simulink library "ddm"  (R2021b)
settings: Solver=VariableStepAuto  StartTime=0.0  StopTime=10.0  RelTol=1e-3
undefined symbols (not defined in the file or in its folder): ENUM_ADASACCSTA_ERROR, ENUM_ADASACCSTA_OFF, ENUM_ADASACCSTA_STANDBY, ENUM_ADASISASTA_OFF, ENUM_ALLOWMOV_ALLOWREADY, ENUM_APS, ENUM_BRKSTA_ERROR, ENUM_BRKSTA_OFF, ENUM_BRKSTA_ON, ENUM_CHGPREACTERRSTA_OBCPRE, ENUM_DCDCFAULTSTA_ANYFAULTLV1, ENUM_DCDCFAULTSTA_ANYFAULTLV2, ENUM_DRIVETRAIN_AWD, ENUM_DRIVETRAIN_FWD, ENUM_DRIVETRAIN_RWD, ENUM_DRSEATSTA_INVALID, ENUM_EDUDRTSTA_NORMAL, ENUM_EPBSTA_APPLIED, ENUM_EPBSTA_RELEASED, ENUM_HVBATTREADYPRE_READY, ENUM_MCUWARN_LV0, ENUM_MCUWARN_LV1, ENUM_MCUWARN_LV2, ENUM_MCUWARN_LV3, ENUM_MCUWARN_NOERROR, ENUM_OBCFAULTSTA_ANYFAULT, ENUM_PAS_R2F2, ENUM_PDFAULT_BATTPDFAIL, ENUM_PDFAULT_DCDCDISABLE, ENUM_PDFAULT_MCUDISABLE, ENUM_PDFAULT_MCUDISCHRG, ENUM_POWERSTA_OFF, ENUM_POWERSTA_ON, ENUM_POWERSTA_READY, ENUM_POWERSTA_STANDBY, ENUM_PRESSINDI_LOW, ENUM_PUFAULT_BATTUPFAIL, ENUM_PUFAULT_DCDCENABLEFAIL, ENUM_PUFAULT_PRECHRGCHKFAIL, ENUM_PUFAULT_SAFETYCHKFAIL, ENUM_PUSTATE_COMPLETED, ENUM_PWRSTASW_OFF, ENUM_PWRSTASW_OFFA, ENUM_PWRSTASW_OFFCHVCHRG, ENUM_PWRSTASW_OFFCLVCHRG, ENUM_PWRSTASW_ON, ENUM_PWRSTASW_ONHVCHRG, ENUM_PWRSTASW_READY, ENUM_PWRSTASW_STANDBY, ENUM_RANGESTA_12IN, ENUM_RANGESTA_12OUT, ENUM_SHIFTCOMMAND_D, ENUM_SHIFTCOMMAND_N, ENUM_SHIFTCOMMAND_P, ENUM_SHIFTCOMMAND_R, ENUM_ZONEMALFUNLV_1ST, ENUM_ZONEMALFUNLV_2ND, ENUM_ZONEMALFUNLV_3RD, ENUM_ZONEMALFUNLV_4TH, ENUM_ZONESPDCTRLMODE_ACC ... (+832)
libraries: hcu_lib x738, $bdroot x26, simulink x7
(part 21 of 25)

== system ddm/DDM/DDM/VMC_DDM/CCU Signal Error/CCU Signal Error  ==
  note: Fail Safe During Detection
  note: Test Detection Criteria
  note: Test Pass Criteria
  note: Release Condiction After Decision
  note: Release Condiction During Detection
  note: Fail Safe After Decision
  note: Diagnostics and Fault Handling
  task_time_s : Inport
  VDDM_C3CCU2LCCFS_flg : Inport  Port=2
  VDDM_C3CCU2RCCFS_flg : Inport  Port=3
  VDDM_C3CCU2CSCFS_flg : Inport  Port=4
  No_CAN_BUS_OFF : Inport  Port=5
  VPMM_PowerSta_enum : Inport  Port=6
  VINP_DCDCFaultSta_enum : Inport  Port=7
  DTC_clear_request : Inport  Port=8
  Constant : Constant  Value=ENUM_POWERSTA_OFF
  Constant1 : Constant  Value=ENUM_POWERSTA_OFF
  Constant{2,10,15,21,23} (5 alike) : Constant  Value=FALSE
  Constant11 : Constant  Value=KDDM_CCUSigErrPassSW_flg
  Constant12 : Constant  Value=ENUM_POWERSTA_OFF
  Constant13 : Constant  Value=ENUM_POWERSTA_STANDBY
  Constant{5,14,18,22} (4 alike) : Constant  Value=TRUE
  Constant3 : Constant  Value=ENUM_DCDCFAULTSTA_ANYFAULTLV2
  Constant33 : Constant  Value=KDDM_CCUSigErrDetSW_flg
  Constant34 : Constant  Value=KDDM_CCUSigErrDTC_cnt
  Constant35 : Constant  Value=KDDM_CCUSigErrCFSSW_flg
  Constant36 : Constant  Value=KDDM_CCUSigErrDFSSW_flg
  Constant4 : Constant  Value=KDDM_CCUSigErrDetTO_ms
  Constant6 : Constant  Value=KDDM_CCUSigErrPassTO_ms
  Constant7 : Constant  Value=KDDM_CCUSigErrDTC_cnt
  Constant8 : Constant  Value=ENUM_DCDCFAULTSTA_ANYFAULTLV2
  Constant9 : Constant  Value=KDDM_CCUSigErrPassTO_ms
  DTC_Couter : hcu_lib/Basic_Blocks/DTC_Couter
  DTC_Info : hcu_lib/Basic_Blocks/DTC_Info
  Data Type Conversion1 : DataTypeConversion  OutDataTypeStr=uint8
  Display1 : Display
  Display2 : Display
  Equal : RelationalOperator  Operator=~=  OutDataTypeStr=boolean  RndMeth=Simplest
  Equal1 : RelationalOperator  Operator=~=  OutDataTypeStr=boolean  RndMeth=Simplest
  Equal{2,4,6..7} (4 alike) : RelationalOperator  Operator===  OutDataTypeStr=boolean  RndMeth=Simplest
  Equal3 : RelationalOperator  OutDataTypeStr=boolean  RndMeth=Simplest
  From1 : From  Commented=on  GotoTag=VDDM_CCUSigErrDFS_flg
  Gain : Gain  Gain=XX2KXX
  Gain1 : Gain  Gain=KXX2XX
  Goto7 : Goto  Commented=on  GotoTag=VDDM_EDriveSysErrVCUErr_flg
  Logical Operator{3,5,9,15,19} (5 alike) : Logic  AllPortsSameDT=off  OutDataTypeStr=boolean
  Logical Operator{6,17..18,20..22,24} (7 alike) : Logic  Operator=NOT  AllPortsSameDT=off  OutDataTypeStr=boolean
  Logical Operator2 : Logic  Inputs=5  AllPortsSameDT=off  OutDataTypeStr=boolean
  Logical Operator23 : Logic  Inputs=5  AllPortsSameDT=off  OutDataTypeStr=boolean
  Logical Operator25 : Logic  Operator=OR  AllPortsSameDT=off  OutDataTypeStr=boolean
  Logical Operator7 : Logic  Operator=OR  AllPortsSameDT=off  OutDataTypeStr=boolean
  Logical Operator8 : Logic  Operator=OR  Inputs=3  AllPortsSameDT=off  OutDataTypeStr=boolean
  Relay : Relay  OnSwitchValue=ONE_INT  OffSwitchValue=ZERO_INT
  SR_Latch1 : hcu_lib/Basic_Blocks/SR_Latch
  SR_Latch4 : hcu_lib/Basic_Blocks/SR_Latch
  SR_Latch5 : hcu_lib/Basic_Blocks/SR_Latch
  Switch{,1..5} (6 alike) : Switch  Criteria=u2 ~= 0
  Terminator1 : Terminator
  Test Detection Criteria : hcu_lib/Basic_Blocks/Test Detection Criteria
  Timer1 : hcu_lib/Basic_Blocks/Timer
  Unit Delay2 : UnitDelay  SampleTime=-1  HasFrameUpgradeWarning=on
  VDDM_CCUSigErrCFS_flg : Outport
  VDDM_CCUSigErrDetDTC_raw32 : Outport  Port=2
  wires:
  Switch2/1 -> [VDDM_xxx_flg], Switch5/3
  Constant23/1 -> Switch1/3
  Constant22/1 -> Switch1/1
  Switch1/1 -> [VDDM_CCUSigErrDFSRls_flg]
  Constant21/1 -> Switch/3
  Switch/1 -> Goto7/1, Display1/1
  Constant18/1 -> Switch/1
  [VDDM_CCUSigErrCFS_flg] -> Switch/2
  [VDDM_CCUSigErrPass_flg] -> Switch1/2
  SR_Latch1/1 -> [VDDM_CCUSigErrPass_flg]
  From1/1 -> Terminator1/1
  [VDDM_CCUSigErrCFS_flg] -> VDDM_CCUSigErrCFS_flg/1
  Constant15/1 -> Switch4/3
  Equal3/1 -> SR_Latch1/1
  [task_time_s] -> Gain1/1
  Equal6/1 -> Logical Operator9/1
  Equal7/1 -> Logical Operator9/2
  Constant6/1 -> Equal3/2
  [VPMM_PowerSta_enum] -> Unit Delay2/1
  Logical Operator9/1 -> Logical Operator8/2
  Switch4/1 -> [VDDM_CCUSigErrCFSRls_flg], Display2/1
  [No_CAN_BUS_OFF] -> Logical Operator2/1
  [VDDM_CCUSigErrPass_flg] -> Logical Operator8/1
  [VDDM_xxx_flg] -> SR_Latch1/2
  [DTC_clear_request] -> Logical Operator8/3
  Logical Operator2/1 -> Switch2/2
  Logical Operator6/1 -> Timer1/1
  Constant13/1 -> Equal7/2
  Constant/1 -> Equal/2
  Unit Delay2/1 -> Equal6/1
  Constant12/1 -> Equal6/2
  Constant2/1 -> Switch2/3
  Constant14/1 -> Switch4/1
  [VPMM_PowerSta_enum] -> Equal7/1
  Logical Operator8/1 -> Switch4/2
  [VPMM_PowerSta_enum] -> Equal/1
  Timer1/1 -> Equal3/1
  VDDM_C3CCU2LCCFS_flg/1 -> [VDDM_C3CCU2LCCFS_flg]
  DTC_clear_request/1 -> [DTC_clear_request]
  VDDM_C3CCU2RCCFS_flg/1 -> [VDDM_C3CCU2RCCFS_flg]
  VPMM_PowerSta_enum/1 -> [VPMM_PowerSta_enum]
  VDDM_C3CCU2CSCFS_flg/1 -> [VDDM_C3CCU2CSCFS_flg]
  No_CAN_BUS_OFF/1 -> [No_CAN_BUS_OFF]
  VINP_DCDCFaultSta_enum/1 -> [VINP_DCDCFaultSta_enum]
  Equal/1 -> Logical Operator2/5
  [VDDM_C3CCU2LCCFS_flg] -> Logical Operator17/1
  [VDDM_C3CCU2RCCFS_flg] -> Logical Operator18/1
  [VDDM_C3CCU2CSCFS_flg] -> Logical Operator20/1
  [VINP_DCDCFaultSta_enum] -> Equal2/1
  Logical Operator17/1 -> Logical Operator2/2
  Logical Operator18/1 -> Logical Operator2/3
  Logical Operator20/1 -> Logical Operator2/4
  Logical Operator22/1 -> Logical Operator23/3
  [VDDM_C3CCU2LCCFS_flg] -> Logical Operator21/1
  [VPMM_PowerSta_enum] -> Equal1/1
  Logical Operator23/1 -> Switch3/2
  Constant5/1 -> Switch3/3
  Equal1/1 -> Logical Operator23/5
  [VDDM_C3CCU2RCCFS_flg] -> Logical Operator22/1
  Logical Operator24/1 -> Logical Operator23/4
  Logical Operator21/1 -> Logical Operator23/2
  [VDDM_C3CCU2CSCFS_flg] -> Logical Operator24/1
  [No_CAN_BUS_OFF] -> Logical Operator23/1
  Constant1/1 -> Equal1/2
  Switch3/1 -> Timer1/2, Logical Operator6/1
  task_time_s/1 -> [task_time_s]  "task_time_s"
  [task_time_s] -> Test Detection Criteria/2
  Constant4/1 -> Gain/1
  Gain/1 -> Test Detection Criteria/4
  Constant7/1 -> Test Detection Criteria/3
  Test Detection Criteria/1 -> [VDDM_CCUSigErrDet_flg]
  Gain1/1 -> Timer1/3
  Constant9/1 -> Timer1/4
  [VDDM_CCUSigErrCFSRls_flg] -> Logical Operator25/2
  [VDDM_CCUSigErrPass_flg] -> Logical Operator25/1
  Logical Operator7/1 -> SR_Latch4/2
  DTC_Couter/2 -> Data Type Conversion1/1
  Relay/1 -> SR_Latch4/1
  Logical Operator3/1 -> [VDDM_CCUSigErrDFS_flg]
  DTC_Couter/1 -> SR_Latch5/1
  Logical Operator25/1 -> Logical Operator15/1
  Constant11/1 -> Logical Operator15/2
  Constant36/1 -> Logical Operator3/1
  Constant34/1 -> DTC_Couter/3
  [VDDM_CCUSigErrDet_flg] -> Logical Operator19/1
  Logical Operator15/1 -> DTC_Couter/2
  Logical Operator19/1 -> DTC_Couter/1
  SR_Latch4/1 -> Logical Operator3/2
  [VDDM_CCUSigErrDTC_cnt] -> Relay/1
  Data Type Conversion1/1 -> [VDDM_CCUSigErrDTC_cnt]
  SR_Latch5/1 -> Logical Operator5/1
  Logical Operator5/1 -> [VDDM_CCUSigErrCFS_flg]
  [VDDM_CCUSigErrCFSRls_flg] -> SR_Latch5/2
  Constant35/1 -> Logical Operator5/2
  [VDDM_CCUSigErrDFSRls_flg] -> Logical Operator7/1
  Constant33/1 -> Logical Operator19/2
  [VDDM_CCUSigErrCFS_flg] -> Logical Operator7/2
  Constant3/1 -> Equal2/2
  Equal2/1 -> Switch2/1
  [VINP_DCDCFaultSta_enum] -> Equal4/1
  Constant8/1 -> Equal4/2
  Equal4/1 -> Switch3/1
  [DTC_clear_request] -> Switch5/2
  Constant10/1 -> Switch5/1
  Switch5/1 -> Test Detection Criteria/1
  [VDDM_CCUSigErrDet_flg] -> DTC_Info/1
  [VDDM_CCUSigErrPass_flg] -> DTC_Info/2
  [VDDM_CCUSigErrCFS_flg] -> DTC_Info/3
  [DTC_clear_request] -> DTC_Info/4
  DTC_Info/1 -> VDDM_CCUSigErrDetDTC_raw32/1  "VDDM_CCUSigErrDetDTC_raw32"

== system ddm/DDM/DDM/VMC_DDM/FCM2/FCM2 Checksum Error  ==
  note: Fail Safe After Decision
  note: Release Condiction During Detection
  note: Diagnostics and Fault Handling
  note: Test Pass Criteria
  note: Release Condiction After Decision
  note: Test Detection Criteria
  note: Fail Safe During Detection
  task_time_s : Inport
  VDDM_FCM2CSErr_flg : Inport  Port=2
  No_CAN_BUS_OFF : Inport  Port=3
  VDDM_FCM2NoComCFS_flg : Inport  Port=4
  VPMM_PowerSta_enum : Inport  Port=5
  VINP_ADASACCSta_enum : Inport  Port=6
  DTC_clear_request : Inport  Port=7
  Constant : Constant  Value=ENUM_POWERSTA_OFF
  Constant{1..2,15,21,23} (5 alike) : Constant  Value=FALSE
  Constant10 : Constant  Value=ENUM_ADASACCSTA_OFF
  Constant11 : Constant  Value=ENUM_ADASACCSTA_STANDBY
  Constant12 : Constant  Value=ENUM_POWERSTA_OFF
  Constant13 : Constant  Value=ENUM_POWERSTA_STANDBY
  Constant{7,14,18,22} (4 alike) : Constant  Value=TRUE
  Constant31 : Constant  Value=KDDM_FCM2CSErrDFSSW_flg
  Constant4 : Constant  Value=KDDM_FCM2CSErrCFSSW_flg
  Constant40 : Constant  Value=KDDM_FCM2CSErrDTC_cnt
  Constant41 : Constant  Value=KDDM_FCM2CSErrDetTO_ms
  Constant45 : Constant  Value=KDDM_FCM2CSErrPassSW_flg
  Constant46 : Constant  Value=KDDM_FCM2CSErrDetSW_flg
  Constant48 : Constant  Value=KDDM_FCM2CSErrDTC_cnt
  Constant5 : Constant  Value=ENUM_POWERSTA_OFF
  Constant6 : Constant  Value=KDDM_FCM2CSErrPassTO_ms
  Constant9 : Constant  Value=KDDM_FCM2CSErrPassTO_ms
  DTC_Couter : hcu_lib/Basic_Blocks/DTC_Couter
  DTC_Info : hcu_lib/Basic_Blocks/DTC_Info
  Data Type Conversion1 : DataTypeConversion  OutDataTypeStr=uint8
  Display : Display
  Display1 : Display
  Display2 : Display
  Equal : RelationalOperator  Operator=~=  OutDataTypeStr=boolean  RndMeth=Simplest
  Equal2 : RelationalOperator  Operator=~=  OutDataTypeStr=boolean  RndMeth=Simplest
  Equal3 : RelationalOperator  OutDataTypeStr=boolean  RndMeth=Simplest
  Equal{4..7} (4 alike) : RelationalOperator  Operator===  OutDataTypeStr=boolean  RndMeth=Simplest
  From6 : From  Commented=on  GotoTag=VDDM_EDriveSysErrVCUErr_flg
  Gain : Gain  Gain=XX2KXX
  Gain1 : Gain  Gain=KXX2XX
  Goto7 : Goto  Commented=on  GotoTag=VDDM_EDriveSysErrVCUErr_flg
  Logical Operator{4..5,9,12,15,18..19} (7 alike) : Logic  AllPortsSameDT=off  OutDataTypeStr=boolean
  Logical Operator16 : Logic  Operator=NOT  AllPortsSameDT=off  OutDataTypeStr=boolean
  Logical Operator2 : Logic  Inputs=3  AllPortsSameDT=off  OutDataTypeStr=boolean
  Logical Operator21 : Logic  Operator=OR  AllPortsSameDT=off  OutDataTypeStr=boolean
  Logical Operator3 : Logic  Operator=OR  AllPortsSameDT=off  OutDataTypeStr=boolean
  Logical Operator6 : Logic  Operator=NOT  AllPortsSameDT=off  OutDataTypeStr=boolean
  Logical Operator7 : Logic  Operator=OR  AllPortsSameDT=off  OutDataTypeStr=boolean
  Logical Operator8 : Logic  Operator=OR  Inputs=3  AllPortsSameDT=off  OutDataTypeStr=boolean
  Relay : Relay  OnSwitchValue=ONE_INT  OffSwitchValue=ZERO_INT
  SR_Latch1 : hcu_lib/Basic_Blocks/SR_Latch
  SR_Latch3 : hcu_lib/Basic_Blocks/SR_Latch
  SR_Latch4 : hcu_lib/Basic_Blocks/SR_Latch
  Switch{,1..5} (6 alike) : Switch  Criteria=u2 ~= 0
  Terminator : Terminator
  Test Detection Criteria : hcu_lib/Basic_Blocks/Test Detection Criteria
  Timer1 : hcu_lib/Basic_Blocks/Timer
  Unit Delay2 : UnitDelay  SampleTime=-1  HasFrameUpgradeWarning=on
  VDDM_FCM2CSErrDFS_flg : Outport
  VDDM_FCM2CSErrCFS_flg : Outport  Port=2
  VDDM_FCM2CSErrDTC_raw32 : Outport  Port=3
  wires:
  VPMM_PowerSta_enum/1 -> [VPMM_PowerSta_enum]
  DTC_clear_request/1 -> [DTC_clear_request]
  No_CAN_BUS_OFF/1 -> [No_CAN_BUS_OFF]
  VINP_ADASACCSta_enum/1 -> [VINP_ADASACCSta_enum]
  VDDM_FCM2CSErr_flg/1 -> [VDDM_FCM2CSErr_flg]
  [VDDM_FCM2CSErrCFS_flg] -> VDDM_FCM2CSErrCFS_flg/1
  [VDDM_FCM2CSErrDFS_flg] -> VDDM_FCM2CSErrDFS_flg/1
  From6/1 -> Terminator/1
  Logical Operator6/1 -> Timer1/1
  Logical Operator21/1 -> SR_Latch3/2
  [VDDM_FCM2CSErrCFS_flg] -> Logical Operator21/2
  Constant22/1 -> Switch1/1
  [VDDM_xxx_flg] -> SR_Latch1/2
  [VDDM_FCM2CSErrCFS_flg] -> Switch/2
  [VINP_ADASACCSta_enum] -> Equal4/1
  [VPMM_PowerSta_enum] -> Unit Delay2/1
  Constant15/1 -> Switch4/3
  [VDDM_FCM2CSErrDTC_cnt] -> Relay/1
  Equal6/1 -> Logical Operator9/1
  Constant13/1 -> Equal7/2
  Constant18/1 -> Switch/1
  Equal3/1 -> SR_Latch1/1
  Switch1/1 -> [VDDM_FCM2CSErrDFSRls_flg]  "VDDM_FCM2CSErrDFSRls_flg"
  Switch/1 -> Display1/1, Goto7/1
  Constant5/1 -> Equal2/2
  [DTC_clear_request] -> Logical Operator8/3
  Unit Delay2/1 -> Equal6/1
  Constant12/1 -> Equal6/2
  Constant2/1 -> Switch2/3
  Logical Operator7/1 -> Logical Operator5/2
  Constant14/1 -> Switch4/1
  Logical Operator4/1 -> Switch3/2
  Equal4/1 -> Logical Operator7/1
  Equal5/1 -> Logical Operator7/2
  Constant7/1 -> Switch3/3
  Logical Operator5/1 -> Logical Operator8/1
  Constant4/1 -> Logical Operator18/2
  [VDDM_FCM2CSErr_flg] -> Switch2/1
  Equal7/1 -> Logical Operator9/2
  [VDDM_FCM2CSErrCFSRls_flg] -> Logical Operator3/2
  Data Type Conversion1/1 -> [VDDM_FCM2CSErrDTC_cnt]  "VDDM_FCM2CSErrDTC_cnt"
  Constant21/1 -> Switch/3
  [VDDM_FCM2CSErrCFSRls_flg] -> SR_Latch4/2
  Constant31/1 -> Logical Operator12/1
  [VDDM_FCM2CSErrPass_flg] -> Switch1/2
  Timer1/1 -> Equal3/1
  Constant23/1 -> Switch1/3
  [VDDM_FCM2CSErrDet_flg] -> Logical Operator19/1
  SR_Latch4/1 -> Logical Operator18/1
  Logical Operator2/1 -> Switch2/2
  Test Detection Criteria/1 -> [VDDM_FCM2CSErrDet_flg]  "VDDM_FCM2CSErrDet_flg"
  [task_time_s] -> Test Detection Criteria/2
  Constant46/1 -> Logical Operator19/2
  [VINP_ADASACCSta_enum] -> Equal5/1
  Logical Operator12/1 -> [VDDM_FCM2CSErrDFS_flg]  "VDDM_FCM2CSErrDFS_flg"
  Constant41/1 -> Gain/1
  [VDDM_FCM2CSErrDFSRls_flg] -> Logical Operator21/1
  Switch4/1 -> Display2/1, [VDDM_FCM2CSErrCFSRls_flg]  "VDDM_FCM2CSErrCFSRls_flg"
  Constant11/1 -> Equal5/2
  [VPMM_PowerSta_enum] -> Equal/1
  Switch3/1 -> Logical Operator6/1, Timer1/2
  Constant/1 -> Equal/2
  DTC_Couter/1 -> SR_Latch4/1
  [VDDM_FCM2CSErrPass_flg] -> Logical Operator3/1
  Constant45/1 -> Logical Operator15/2
  Logical Operator19/1 -> DTC_Couter/1
  [VDDM_FCM2CSErr_flg] -> Switch3/1
  [VPMM_PowerSta_enum] -> Equal2/1
  [VPMM_PowerSta_enum] -> Equal7/1
  Logical Operator8/1 -> Switch4/2
  Logical Operator9/1 -> Logical Operator8/2
  [No_CAN_BUS_OFF] -> Logical Operator4/1
  Constant10/1 -> Equal4/2
  Constant48/1 -> DTC_Couter/3
  Equal2/1 -> Logical Operator4/2
  [VDDM_FCM2CSErrPass_flg] -> Logical Operator5/1
  Logical Operator3/1 -> Logical Operator15/1
  Relay/1 -> SR_Latch3/1
  Logical Operator18/1 -> [VDDM_FCM2CSErrCFS_flg]  "VDDM_FCM2CSErrCFS_flg"
  Equal/1 -> Logical Operator2/3
  Gain/1 -> Test Detection Criteria/4
  SR_Latch1/1 -> Display/1, [VDDM_FCM2CSErrPass_flg]  "VDDM_FCM2CSErrPass_flg"
  Constant6/1 -> Equal3/2
  Logical Operator15/1 -> DTC_Couter/2
  SR_Latch3/1 -> Logical Operator12/2
  Constant40/1 -> Test Detection Criteria/3
  DTC_Couter/2 -> Data Type Conversion1/1
  task_time_s/1 -> [task_time_s]  "task_time_s"
  Constant9/1 -> Timer1/4
  [VDDM_FCM2NoComCFS_flg] -> Logical Operator16/1
  Logical Operator16/1 -> Logical Operator2/2
  [No_CAN_BUS_OFF] -> Logical Operator2/1
  VDDM_FCM2NoComCFS_flg/1 -> [VDDM_FCM2NoComCFS_flg]
  [task_time_s] -> Gain1/1
  Gain1/1 -> Timer1/3
  Switch2/1 -> [VDDM_xxx_flg], Switch5/3
  Constant1/1 -> Switch5/1
  [DTC_clear_request] -> Switch5/2
  Switch5/1 -> Test Detection Criteria/1
  [VDDM_FCM2CSErrDet_flg] -> DTC_Info/1
  [VDDM_FCM2CSErrPass_flg] -> DTC_Info/2
  [VDDM_FCM2CSErrCFS_flg] -> DTC_Info/3
  [DTC_clear_request] -> DTC_Info/4
  DTC_Info/1 -> VDDM_FCM2CSErrDTC_raw32/1  "VDDM_FCM2CSErrDTC_raw32"

== system ddm/DDM/DDM/VMC_DDM/FCM2/FCM2 Lost Com ==
  note: Fail Safe After Decision
  note: Release Condiction During Detection
  note: Diagnostics and Fault Handling
  note: Test Pass Criteria
  note: Release Condiction After Decision
  note: Test Detection Criteria
  note: Fail Safe During Detection
  task_time_s : Inport
  VDDM_FCM2NoCom_flg : Inport  Port=2
  No_CAN_BUS_OFF : Inport  Port=3
  VPMM_PowerSta_enum : Inport  Port=4
  VINP_ADASACCSta_enum : Inport  Port=5
  DTC_clear_request : Inport  Port=6
  Constant : Constant  Value=ENUM_POWERSTA_OFF
  Constant{1..2,15,21,23} (5 alike) : Constant  Value=FALSE
  Constant10 : Constant  Value=ENUM_ADASACCSTA_OFF
  Constant11 : Constant  Value=ENUM_ADASACCSTA_STANDBY
  Constant12 : Constant  Value=ENUM_POWERSTA_OFF
  Constant13 : Constant  Value=ENUM_POWERSTA_STANDBY
  Constant{7,14,18,22} (4 alike) : Constant  Value=TRUE
  Constant31 : Constant  Value=KDDM_FCM2NoComDFSSW_flg
  Constant4 : Constant  Value=KDDM_FCM2NoComCFSSW_flg
  Constant40 : Constant  Value=KDDM_FCM2NoComDTC_cnt
  Constant41 : Constant  Value=KDDM_FCM2NoComDetTO_ms
  Constant45 : Constant  Value=KDDM_FCM2NoComPassSW_flg
  Constant46 : Constant  Value=KDDM_FCM2NoComDetSW_flg
  Constant48 : Constant  Value=KDDM_FCM2NoComDTC_cnt
  Constant5 : Constant  Value=ENUM_POWERSTA_OFF
  Constant6 : Constant  Value=KDDM_FCM2NoComPassTO_ms
  Constant9 : Constant  Value=KDDM_FCM2NoComPassTO_ms
  DTC_Couter : hcu_lib/Basic_Blocks/DTC_Couter
  DTC_Info : hcu_lib/Basic_Blocks/DTC_Info
  Data Type Conversion1 : DataTypeConversion  OutDataTypeStr=uint8
  Display : Display
  Display1 : Display
  Display2 : Display
  Equal : RelationalOperator  Operator=~=  OutDataTypeStr=boolean  RndMeth=Simplest
  Equal2 : RelationalOperator  Operator=~=  OutDataTypeStr=boolean  RndMeth=Simplest
  Equal3 : RelationalOperator  OutDataTypeStr=boolean  RndMeth=Simplest
  Equal{4..7} (4 alike) : RelationalOperator  Operator===  OutDataTypeStr=boolean  RndMeth=Simplest
  From6 : From  Commented=on  GotoTag=VDDM_EDriveSysErrVCUErr_flg
  Gain : Gain  Gain=XX2KXX
  Gain1 : Gain  Gain=KXX2XX
  Goto7 : Goto  Commented=on  GotoTag=VDDM_EDriveSysErrVCUErr_flg
  Logical Operator{2,4..5,9,12,15,18..19} (8 alike) : Logic  AllPortsSameDT=off  OutDataTypeStr=boolean
  Logical Operator21 : Logic  Operator=OR  AllPortsSameDT=off  OutDataTypeStr=boolean
  Logical Operator3 : Logic  Operator=OR  AllPortsSameDT=off  OutDataTypeStr=boolean
  Logical Operator6 : Logic  Operator=NOT  AllPortsSameDT=off  OutDataTypeStr=boolean
  Logical Operator7 : Logic  Operator=OR  AllPortsSameDT=off  OutDataTypeStr=boolean
  Logical Operator8 : Logic  Operator=OR  Inputs=3  AllPortsSameDT=off  OutDataTypeStr=boolean
  Relay : Relay  OnSwitchValue=ONE_INT  OffSwitchValue=ZERO_INT
  SR_Latch1 : hcu_lib/Basic_Blocks/SR_Latch
  SR_Latch3 : hcu_lib/Basic_Blocks/SR_Latch
  SR_Latch4 : hcu_lib/Basic_Blocks/SR_Latch
  Switch{,1..5} (6 alike) : Switch  Criteria=u2 ~= 0
  Terminator : Terminator
  Test Detection Criteria : hcu_lib/Basic_Blocks/Test Detection Criteria
  Timer1 : hcu_lib/Basic_Blocks/Timer
  Unit Delay2 : UnitDelay  SampleTime=-1  HasFrameUpgradeWarning=on
  VDDM_FCM2NoComDFS_flg : Outport
  VDDM_FCM2NoComCFS_flg : Outport  Port=2
  VDDM_FCM2NoComDTC_raw32 : Outport  Port=3
  wires:
  VPMM_PowerSta_enum/1 -> [VPMM_PowerSta_enum]
  DTC_clear_request/1 -> [DTC_clear_request]
  No_CAN_BUS_OFF/1 -> [No_CAN_BUS_OFF]
  VINP_ADASACCSta_enum/1 -> [VINP_ADASACCSta_enum]
  VDDM_FCM2NoCom_flg/1 -> [VDDM_FCM2NoCom_flg]
  [VDDM_FCM2NoComCFS_flg] -> VDDM_FCM2NoComCFS_flg/1
  [VDDM_FCM2NoComDFS_flg] -> VDDM_FCM2NoComDFS_flg/1
  From6/1 -> Terminator/1
  Logical Operator6/1 -> Timer1/1
  Logical Operator21/1 -> SR_Latch3/2
  [VDDM_FCM2NoComCFS_flg] -> Logical Operator21/2
  Constant22/1 -> Switch1/1
  [VDDM_xxx_flg] -> SR_Latch1/2
  [No_CAN_BUS_OFF] -> Logical Operator2/1
  [VDDM_FCM2NoComCFS_flg] -> Switch/2
  [VINP_ADASACCSta_enum] -> Equal4/1
  [VPMM_PowerSta_enum] -> Unit Delay2/1
  Constant15/1 -> Switch4/3
  [VDDM_FCM2NoComDTC_cnt] -> Relay/1
  [task_time_s] -> Gain1/1
  Equal6/1 -> Logical Operator9/1
  Constant13/1 -> Equal7/2
  Constant18/1 -> Switch/1
  Equal3/1 -> SR_Latch1/1
  Switch1/1 -> [VDDM_FCM2NoComDFSRls_flg]  "VDDM_FCM2NoComDFSRls_flg"
  Switch/1 -> Display1/1, Goto7/1
  Constant5/1 -> Equal2/2
  [DTC_clear_request] -> Logical Operator8/3
  Unit Delay2/1 -> Equal6/1
  Constant12/1 -> Equal6/2
  Constant2/1 -> Switch2/3
  Logical Operator7/1 -> Logical Operator5/2
  Constant14/1 -> Switch4/1
  Logical Operator4/1 -> Switch3/2
  Equal4/1 -> Logical Operator7/1
  Equal5/1 -> Logical Operator7/2
  Constant7/1 -> Switch3/3
  Logical Operator5/1 -> Logical Operator8/1
  Constant4/1 -> Logical Operator18/2
  [VDDM_FCM2NoCom_flg] -> Switch2/1
  Equal7/1 -> Logical Operator9/2
  [VDDM_FCM2NoComCFSRls_flg] -> Logical Operator3/2
  Data Type Conversion1/1 -> [VDDM_FCM2NoComDTC_cnt]  "VDDM_FCM2NoComDTC_cnt"
  Constant21/1 -> Switch/3
  [VDDM_FCM2NoComCFSRls_flg] -> SR_Latch4/2
  Constant31/1 -> Logical Operator12/1
  [VDDM_FCM2NoComPass_flg] -> Switch1/2
  Timer1/1 -> Equal3/1
  Constant23/1 -> Switch1/3
  [VDDM_FCM2NoComDet_flg] -> Logical Operator19/1
  SR_Latch4/1 -> Logical Operator18/1
  Logical Operator2/1 -> Switch2/2
  Test Detection Criteria/1 -> [VDDM_FCM2NoComDet_flg]  "VDDM_FCM2NoComDet_flg"
  [task_time_s] -> Test Detection Criteria/2
  Constant46/1 -> Logical Operator19/2
  [VINP_ADASACCSta_enum] -> Equal5/1
  Logical Operator12/1 -> [VDDM_FCM2NoComDFS_flg]  "VDDM_FCM2NoComDFS_flg"
  Constant41/1 -> Gain/1
  [VDDM_FCM2NoComDFSRls_flg] -> Logical Operator21/1
  Switch4/1 -> Display2/1, [VDDM_FCM2NoComCFSRls_flg]  "VDDM_FCM2NoComCFSRls_flg"
  Constant11/1 -> Equal5/2
  [VPMM_PowerSta_enum] -> Equal/1
  Switch3/1 -> Logical Operator6/1, Timer1/2
  Constant/1 -> Equal/2
  DTC_Couter/1 -> SR_Latch4/1
  Switch2/1 -> [VDDM_xxx_flg], Switch5/3
  [VDDM_FCM2NoComPass_flg] -> Logical Operator3/1
  Constant45/1 -> Logical Operator15/2
  Logical Operator19/1 -> DTC_Couter/1
  [VDDM_FCM2NoCom_flg] -> Switch3/1
  [VPMM_PowerSta_enum] -> Equal2/1
  [VPMM_PowerSta_enum] -> Equal7/1
  Logical Operator8/1 -> Switch4/2
  Logical Operator9/1 -> Logical Operator8/2
  [No_CAN_BUS_OFF] -> Logical Operator4/1
  Constant10/1 -> Equal4/2
  Constant48/1 -> DTC_Couter/3
  Equal2/1 -> Logical Operator4/2
  [VDDM_FCM2NoComPass_flg] -> Logical Operator5/1
  Logical Operator3/1 -> Logical Operator15/1
  Relay/1 -> SR_Latch3/1
  Logical Operator18/1 -> [VDDM_FCM2NoComCFS_flg]  "VDDM_FCM2NoComCFS_flg"
  Equal/1 -> Logical Operator2/2
  Gain/1 -> Test Detection Criteria/4
  SR_Latch1/1 -> Display/1, [VDDM_FCM2NoComPass_flg]  "VDDM_FCM2NoComPass_flg"
  Constant6/1 -> Equal3/2
  Logical Operator15/1 -> DTC_Couter/2
  SR_Latch3/1 -> Logical Operator12/2
  Constant40/1 -> Test Detection Criteria/3
  DTC_Couter/2 -> Data Type Conversion1/1
  task_time_s/1 -> [task_time_s]  "task_time_s"
  Constant9/1 -> Timer1/4
  Gain1/1 -> Timer1/3
  Switch5/1 -> Test Detection Criteria/1
  [DTC_clear_request] -> Switch5/2
  Constant1/1 -> Switch5/1
  [VDDM_FCM2NoComDet_flg] -> DTC_Info/1
  [VDDM_FCM2NoComPass_flg] -> DTC_Info/2
  [VDDM_FCM2NoComCFS_flg] -> DTC_Info/3
  [DTC_clear_request] -> DTC_Info/4
  DTC_Info/1 -> VDDM_FCM2NoComDTC_raw32/1  "VDDM_FCM2NoComDTC_raw32"

== system ddm/DDM/DDM/VMC_DDM/FCM2/FCM2 Rolling Count Error  ==
  note: Fail Safe After Decision
  note: Release Condiction During Detection
  note: Diagnostics and Fault Handling
  note: Test Pass Criteria
  note: Release Condiction After Decision
  note: Test Detection Criteria
  note: Fail Safe During Detection
  task_time_s : Inport
  VDDM_FCM2RCErr_flg : Inport  Port=2
  No_CAN_BUS_OFF : Inport  Port=3
  VDDM_FCM2NoComCFS_flg : Inport  Port=4
  VPMM_PowerSta_enum : Inport  Port=5
  VINP_ADASACCSta_enum : Inport  Port=6
  DTC_clear_request : Inport  Port=7
  Constant : Constant  Value=ENUM_POWERSTA_OFF
  Constant{1..2,15,21,23} (5 alike) : Constant  Value=FALSE
  Constant10 : Constant  Value=ENUM_ADASACCSTA_OFF
  Constant11 : Constant  Value=ENUM_ADASACCSTA_STANDBY
  Constant12 : Constant  Value=ENUM_POWERSTA_OFF
  Constant13 : Constant  Value=ENUM_POWERSTA_STANDBY
  Constant{7,14,18,22} (4 alike) : Constant  Value=TRUE
  Constant31 : Constant  Value=KDDM_FCM2RCErrDFSSW_flg
  Constant4 : Constant  Value=KDDM_FCM2RCErrCFSSW_flg
  Constant40 : Constant  Value=KDDM_FCM2RCErrDTC_cnt
  Constant41 : Constant  Value=KDDM_FCM2RCErrDetTO_ms
  Constant45 : Constant  Value=KDDM_FCM2RCErrPassSW_flg
  Constant46 : Constant  Value=KDDM_FCM2RCErrDetSW_flg
  Constant48 : Constant  Value=KDDM_FCM2RCErrDTC_cnt
  Constant5 : Constant  Value=ENUM_POWERSTA_OFF
  Constant6 : Constant  Value=KDDM_FCM2RCErrPassTO_ms
  Constant9 : Constant  Value=KDDM_FCM2RCErrPassTO_ms
  DTC_Couter : hcu_lib/Basic_Blocks/DTC_Couter
  DTC_Info : hcu_lib/Basic_Blocks/DTC_Info
  Data Type Conversion1 : DataTypeConversion  OutDataTypeStr=uint8
  Display : Display
  Display1 : Display
  Display2 : Display
  Equal : RelationalOperator  Operator=~=  OutDataTypeStr=boolean  RndMeth=Simplest
  Equal2 : RelationalOperator  Operator=~=  OutDataTypeStr=boolean  RndMeth=Simplest
  Equal3 : RelationalOperator  OutDataTypeStr=boolean  RndMeth=Simplest
  Equal{4..7} (4 alike) : RelationalOperator  Operator===  OutDataTypeStr=boolean  RndMeth=Simplest
  From6 : From  Commented=on  GotoTag=VDDM_EDriveSysErrVCUErr_flg
  Gain : Gain  Gain=XX2KXX
  Gain1 : Gain  Gain=KXX2XX
  Goto7 : Goto  Commented=on  GotoTag=VDDM_EDriveSysErrVCUErr_flg
  Logical Operator{4..5,9,12,15,18..19} (7 alike) : Logic  AllPortsSameDT=off  OutDataTypeStr=boolean
  Logical Operator16 : Logic  Operator=NOT  AllPortsSameDT=off  OutDataTypeStr=boolean
  Logical Operator2 : Logic  Inputs=3  AllPortsSameDT=off  OutDataTypeStr=boolean
  Logical Operator21 : Logic  Operator=OR  AllPortsSameDT=off  OutDataTypeStr=boolean
  Logical Operator3 : Logic  Operator=OR  AllPortsSameDT=off  OutDataTypeStr=boolean
  Logical Operator6 : Logic  Operator=NOT  AllPortsSameDT=off  OutDataTypeStr=boolean
  Logical Operator7 : Logic  Operator=OR  AllPortsSameDT=off  OutDataTypeStr=boolean
  Logical Operator8 : Logic  Operator=OR  Inputs=3  AllPortsSameDT=off  OutDataTypeStr=boolean
  Relay : Relay  OnSwitchValue=ONE_INT  OffSwitchValue=ZERO_INT
  SR_Latch1 : hcu_lib/Basic_Blocks/SR_Latch
  SR_Latch3 : hcu_lib/Basic_Blocks/SR_Latch
  SR_Latch4 : hcu_lib/Basic_Blocks/SR_Latch
  Switch{,1..5} (6 alike) : Switch  Criteria=u2 ~= 0
  Terminator : Terminator
  Test Detection Criteria : hcu_lib/Basic_Blocks/Test Detection Criteria
  Timer1 : hcu_lib/Basic_Blocks/Timer
  Unit Delay2 : UnitDelay  SampleTime=-1  HasFrameUpgradeWarning=on
  VDDM_FCM2RCErrDFS_flg : Outport
  VDDM_FCM2RCErrCFS_flg : Outport  Port=2
  VDDM_FCM2RCErrDTC_raw32 : Outport  Port=3
  wires:
  VPMM_PowerSta_enum/1 -> [VPMM_PowerSta_enum]
  DTC_clear_request/1 -> [DTC_clear_request]
  No_CAN_BUS_OFF/1 -> [No_CAN_BUS_OFF]
  VINP_ADASACCSta_enum/1 -> [VINP_ADASACCSta_enum]
  VDDM_FCM2RCErr_flg/1 -> [VDDM_FCM2RCErr_flg]
  [VDDM_FCM2RCErrCFS_flg] -> VDDM_FCM2RCErrCFS_flg/1
  [VDDM_FCM2RCErrDFS_flg] -> VDDM_FCM2RCErrDFS_flg/1
  From6/1 -> Terminator/1
  Logical Operator6/1 -> Timer1/1
  Logical Operator21/1 -> SR_Latch3/2
  [VDDM_FCM2RCErrCFS_flg] -> Logical Operator21/2
  Constant22/1 -> Switch1/1
  [VDDM_xxx_flg] -> SR_Latch1/2
  [VDDM_FCM2RCErrCFS_flg] -> Switch/2
  [VINP_ADASACCSta_enum] -> Equal4/1
  [VPMM_PowerSta_enum] -> Unit Delay2/1
  Constant15/1 -> Switch4/3
  [VDDM_FCM2RCErrDTC_cnt] -> Relay/1
  Equal6/1 -> Logical Operator9/1
  Constant13/1 -> Equal7/2
  Constant18/1 -> Switch/1
  Equal3/1 -> SR_Latch1/1
  Switch1/1 -> [VDDM_FCM2RCErrDFSRls_flg]  "VDDM_FCM2RCErrDFSRls_flg"
  Switch/1 -> Display1/1, Goto7/1
  Constant5/1 -> Equal2/2
  [DTC_clear_request] -> Logical Operator8/3
  Unit Delay2/1 -> Equal6/1
  Constant12/1 -> Equal6/2
  Constant2/1 -> Switch2/3
  Logical Operator7/1 -> Logical Operator5/2
  Constant14/1 -> Switch4/1
  Logical Operator4/1 -> Switch3/2
  Equal4/1 -> Logical Operator7/1
  Equal5/1 -> Logical Operator7/2
  Constant7/1 -> Switch3/3
  Logical Operator5/1 -> Logical Operator8/1
  Constant4/1 -> Logical Operator18/2
  [VDDM_FCM2RCErr_flg] -> Switch2/1
  Equal7/1 -> Logical Operator9/2
  [VDDM_FCM2RCErrCFSRls_flg] -> Logical Operator3/2
  Data Type Conversion1/1 -> [VDDM_FCM2RCErrDTC_cnt]  "VDDM_FCM2RCErrDTC_cnt"
  Constant21/1 -> Switch/3
  [VDDM_FCM2RCErrCFSRls_flg] -> SR_Latch4/2
  Constant31/1 -> Logical Operator12/1
  [VDDM_FCM2RCErrPass_flg] -> Switch1/2
  Timer1/1 -> Equal3/1
  Constant23/1 -> Switch1/3
  [VDDM_FCM2RCErrDet_flg] -> Logical Operator19/1
  SR_Latch4/1 -> Logical Operator18/1
  Logical Operator2/1 -> Switch2/2
  Test Detection Criteria/1 -> [VDDM_FCM2RCErrDet_flg]  "VDDM_FCM2RCErrDet_flg"
  [task_time_s] -> Test Detection Criteria/2
  Constant46/1 -> Logical Operator19/2
  [VINP_ADASACCSta_enum] -> Equal5/1
  Logical Operator12/1 -> [VDDM_FCM2RCErrDFS_flg]  "VDDM_FCM2RCErrDFS_flg"
  Constant41/1 -> Gain/1
  [VDDM_FCM2RCErrDFSRls_flg] -> Logical Operator21/1
  Switch4/1 -> Display2/1, [VDDM_FCM2RCErrCFSRls_flg]  "VDDM_FCM2RCErrCFSRls_flg"
  Constant11/1 -> Equal5/2
  [VPMM_PowerSta_enum] -> Equal/1
  Switch3/1 -> Logical Operator6/1, Timer1/2
  Constant/1 -> Equal/2
  DTC_Couter/1 -> SR_Latch4/1
  Switch2/1 -> [VDDM_xxx_flg], Switch5/3
  [VDDM_FCM2RCErrPass_flg] -> Logical Operator3/1
  Constant45/1 -> Logical Operator15/2
  Logical Operator19/1 -> DTC_Couter/1
  [VDDM_FCM2RCErr_flg] -> Switch3/1
  [VPMM_PowerSta_enum] -> Equal2/1
  [VPMM_PowerSta_enum] -> Equal7/1
  Logical Operator8/1 -> Switch4/2
  Logical Operator9/1 -> Logical Operator8/2
  [No_CAN_BUS_OFF] -> Logical Operator4/1
  Constant10/1 -> Equal4/2
  Constant48/1 -> DTC_Couter/3
  Equal2/1 -> Logical Operator4/2
  [VDDM_FCM2RCErrPass_flg] -> Logical Operator5/1
  Logical Operator3/1 -> Logical Operator15/1
  Relay/1 -> SR_Latch3/1
  Logical Operator18/1 -> [VDDM_FCM2RCErrCFS_flg]  "VDDM_FCM2RCErrCFS_flg"
  Equal/1 -> Logical Operator2/3
  Gain/1 -> Test Detection Criteria/4
  SR_Latch1/1 -> Display/1, [VDDM_FCM2RCErrPass_flg]  "VDDM_FCM2RCErrPass_flg"
  Constant6/1 -> Equal3/2
  Logical Operator15/1 -> DTC_Couter/2
  SR_Latch3/1 -> Logical Operator12/2
  Constant40/1 -> Test Detection Criteria/3
  DTC_Couter/2 -> Data Type Conversion1/1
  task_time_s/1 -> [task_time_s]  "task_time_s"
  Constant9/1 -> Timer1/4
  [VDDM_FCM2NoComCFS_flg] -> Logical Operator16/1
  Logical Operator16/1 -> Logical Operator2/2
  [No_CAN_BUS_OFF] -> Logical Operator2/1
  VDDM_FCM2NoComCFS_flg/1 -> [VDDM_FCM2NoComCFS_flg]
  Gain1/1 -> Timer1/3
  [task_time_s] -> Gain1/1
  [DTC_clear_request] -> Switch5/2
  Constant1/1 -> Switch5/1
  Switch5/1 -> Test Detection Criteria/1
  [VDDM_FCM2RCErrDet_flg] -> DTC_Info/1
  [VDDM_FCM2RCErrPass_flg] -> DTC_Info/2
  [VDDM_FCM2RCErrCFS_flg] -> DTC_Info/3
  [DTC_clear_request] -> DTC_Info/4
  DTC_Info/1 -> VDDM_FCM2RCErrDTC_raw32/1  "VDDM_FCM2RCErrDTC_raw32"

== system ddm/DDM/DDM/VMC_DDM/FCM3/FCM3 Checksum Error  ==
  note: Fail Safe After Decision
  note: Release Condiction During Detection
  note: Diagnostics and Fault Handling
  note: Test Pass Criteria
  note: Release Condiction After Decision
  note: Test Detection Criteria
  note: Fail Safe During Detection
  task_time_s : Inport
  VDDM_FCM3CSErr_flg : Inport  Port=2
  No_CAN_BUS_OFF : Inport  Port=3
  VDDM_FCM3NoComCFS_flg : Inport  Port=4
  VPMM_PowerSta_enum : Inport  Port=5
  VINP_ADASACCSta_enum : Inport  Port=6
  VINP_ADASISASta_enum : Inport  Port=7
  DTC_clear_request : Inport  Port=8
  Constant : Constant  Value=ENUM_POWERSTA_OFF
  Constant1 : Constant  Value=ENUM_ADASACCSTA_OFF
  Constant{2,10,15,21,23} (5 alike) : Constant  Value=FALSE
  Constant{7,14,18,22} (4 alike) : Constant  Value=TRUE
  Constant16 : Constant  Value=ENUM_POWERSTA_STANDBY
  Constant17 : Constant  Value=ENUM_ADASISASTA_OFF
  Constant3 : Constant  Value=ENUM_ADASACCSTA_STANDBY
  Constant31 : Constant  Value=KDDM_FCM3CSErrDFSSW_flg
  Constant4 : Constant  Value=KDDM_FCM3CSErrCFSSW_flg
  Constant40 : Constant  Value=KDDM_FCM3CSErrDTC_cnt
  Constant41 : Constant  Value=KDDM_FCM3CSErrDetTO_ms
  Constant45 : Constant  Value=KDDM_FCM3CSErrPassSW_flg
  Constant46 : Constant  Value=KDDM_FCM3CSErrDetSW_flg
  Constant48 : Constant  Value=KDDM_FCM3CSErrDTC_cnt
  Constant5 : Constant  Value=ENUM_POWERSTA_OFF
  Constant6 : Constant  Value=KDDM_FCM3CSErrPassTO_ms
  Constant8 : Constant  Value=ENUM_POWERSTA_OFF
  Constant9 : Constant  Value=KDDM_FCM3CSErrPassTO_ms
  DTC_Couter : hcu_lib/Basic_Blocks/DTC_Couter
  DTC_Info : hcu_lib/Basic_Blocks/DTC_Info
  Data Type Conversion1 : DataTypeConversion  OutDataTypeStr=uint8
  Display : Display
  Display1 : Display
  Display2 : Display
  Equal : RelationalOperator  Operator=~=  OutDataTypeStr=boolean  RndMeth=Simplest
  Equal{1,8..11} (5 alike) : RelationalOperator  Operator===  OutDataTypeStr=boolean  RndMeth=Simplest
  Equal2 : RelationalOperator  Operator=~=  OutDataTypeStr=boolean  RndMeth=Simplest
  Equal3 : RelationalOperator  OutDataTypeStr=boolean  RndMeth=Simplest
  From6 : From  Commented=on  GotoTag=VDDM_EDriveSysErrVCUErr_flg
  Gain : Gain  Gain=XX2KXX
  Gain1 : Gain  Gain=KXX2XX
  Goto7 : Goto  Commented=on  GotoTag=VDDM_EDriveSysErrVCUErr_flg
  Logical Operator1 : Logic  Inputs=3  AllPortsSameDT=off  OutDataTypeStr=boolean
  Logical Operator10 : Logic  Operator=OR  AllPortsSameDT=off  OutDataTypeStr=boolean
  Logical Operator11 : Logic  Operator=OR  Inputs=3  AllPortsSameDT=off  OutDataTypeStr=boolean
  Logical Operator{4,12..13,15,18..19} (6 alike) : Logic  AllPortsSameDT=off  OutDataTypeStr=boolean
  Logical Operator16 : Logic  Operator=NOT  AllPortsSameDT=off  OutDataTypeStr=boolean
  Logical Operator2 : Logic  Inputs=3  AllPortsSameDT=off  OutDataTypeStr=boolean
  Logical Operator21 : Logic  Operator=OR  AllPortsSameDT=off  OutDataTypeStr=boolean
  Logical Operator3 : Logic  Operator=OR  AllPortsSameDT=off  OutDataTypeStr=boolean
  Logical Operator6 : Logic  Operator=NOT  AllPortsSameDT=off  OutDataTypeStr=boolean
  Relay : Relay  OnSwitchValue=ONE_INT  OffSwitchValue=ZERO_INT
  SR_Latch1 : hcu_lib/Basic_Blocks/SR_Latch
  SR_Latch3 : hcu_lib/Basic_Blocks/SR_Latch
  SR_Latch4 : hcu_lib/Basic_Blocks/SR_Latch
  Switch{,1..5} (6 alike) : Switch  Criteria=u2 ~= 0
  Terminator : Terminator
  Test Detection Criteria : hcu_lib/Basic_Blocks/Test Detection Criteria
  Timer1 : hcu_lib/Basic_Blocks/Timer
  Unit Delay1 : UnitDelay  SampleTime=-1  HasFrameUpgradeWarning=on
  VDDM_FCM3CSErrDFS_flg : Outport
  VDDM_FCM3CSErrCFS_flg : Outport  Port=2
  VDDM_FCM3CSErrDTC_raw32 : Outport  Port=3
  wires:
  VPMM_PowerSta_enum/1 -> [VPMM_PowerSta_enum]
  DTC_clear_request/1 -> [DTC_clear_request]
  No_CAN_BUS_OFF/1 -> [No_CAN_BUS_OFF]
  VINP_ADASACCSta_enum/1 -> [VINP_ADASACCSta_enum]
  VDDM_FCM3CSErr_flg/1 -> [VDDM_FCM3CSErr_flg]
  [VDDM_FCM3CSErrCFS_flg] -> VDDM_FCM3CSErrCFS_flg/1
  [VDDM_FCM3CSErrDFS_flg] -> VDDM_FCM3CSErrDFS_flg/1
  From6/1 -> Terminator/1
  Logical Operator6/1 -> Timer1/1
  Logical Operator21/1 -> SR_Latch3/2
  [VDDM_FCM3CSErrCFS_flg] -> Logical Operator21/2
  Constant22/1 -> Switch1/1
  [VDDM_xxx_flg] -> SR_Latch1/2
  [VDDM_FCM3CSErrCFS_flg] -> Switch/2
  Constant15/1 -> Switch4/3
  [VDDM_FCM3CSErrDTC_cnt] -> Relay/1
  Constant18/1 -> Switch/1
  Equal3/1 -> SR_Latch1/1
  Switch1/1 -> [VDDM_FCM3CSErrDFSRls_flg]
  Switch/1 -> Display1/1, Goto7/1
  Constant5/1 -> Equal2/2
  Constant2/1 -> Switch2/3
  Constant14/1 -> Switch4/1
  Logical Operator4/1 -> Switch3/2
  Constant7/1 -> Switch3/3
  Constant4/1 -> Logical Operator18/2
  [VDDM_FCM3CSErr_flg] -> Switch2/1
  [VDDM_FCM3CSErrCFSRls_flg] -> Logical Operator3/2
  Data Type Conversion1/1 -> [VDDM_FCM3CSErrDTC_cnt]
  Constant21/1 -> Switch/3
  [VDDM_FCM3CSErrCFSRls_flg] -> SR_Latch4/2
  Constant31/1 -> Logical Operator12/1
  [VDDM_FCM3CSErrPass_flg] -> Switch1/2
  Timer1/1 -> Equal3/1
  Constant23/1 -> Switch1/3
  [VDDM_FCM3CSErrDet_flg] -> Logical Operator19/1
  SR_Latch4/1 -> Logical Operator18/1
  Logical Operator2/1 -> Switch2/2
  Test Detection Criteria/1 -> [VDDM_FCM3CSErrDet_flg]
  [task_time_s] -> Test Detection Criteria/2
  Constant46/1 -> Logical Operator19/2
  Logical Operator12/1 -> [VDDM_FCM3CSErrDFS_flg]
  Constant41/1 -> Gain/1
  [VDDM_FCM3CSErrDFSRls_flg] -> Logical Operator21/1
  Switch4/1 -> Display2/1, [VDDM_FCM3CSErrCFSRls_flg]
  [VPMM_PowerSta_enum] -> Equal/1
  Switch3/1 -> Logical Operator6/1, Timer1/2
  Constant/1 -> Equal/2
  DTC_Couter/1 -> SR_Latch4/1
  Switch2/1 -> [VDDM_xxx_flg], Switch5/3
  [VDDM_FCM3CSErrPass_flg] -> Logical Operator3/1
  Constant45/1 -> Logical Operator15/2
  Logical Operator19/1 -> DTC_Couter/1
  [VDDM_FCM3CSErr_flg] -> Switch3/1
  [VPMM_PowerSta_enum] -> Equal2/1
  [No_CAN_BUS_OFF] -> Logical Operator4/1
  Constant48/1 -> DTC_Couter/3
  Equal2/1 -> Logical Operator4/2
  [VDDM_FCM3CSErrPass_flg] -> Logical Operator1/1
  Logical Operator3/1 -> Logical Operator15/1
  Relay/1 -> SR_Latch3/1
  Logical Operator18/1 -> [VDDM_FCM3CSErrCFS_flg]
  Equal/1 -> Logical Operator2/3
  Gain/1 -> Test Detection Criteria/4
  SR_Latch1/1 -> Display/1, [VDDM_FCM3CSErrPass_flg]
  Constant6/1 -> Equal3/2
  Logical Operator15/1 -> DTC_Couter/2
  SR_Latch3/1 -> Logical Operator12/2
  Constant40/1 -> Test Detection Criteria/3
  DTC_Couter/2 -> Data Type Conversion1/1
  task_time_s/1 -> [task_time_s]  "task_time_s"
  Constant9/1 -> Timer1/4
  [VDDM_FCM3NoComCFS_flg] -> Logical Operator16/1
  Logical Operator16/1 -> Logical Operator2/2
  [No_CAN_BUS_OFF] -> Logical Operator2/1
  VDDM_FCM3NoComCFS_flg/1 -> [VDDM_FCM3NoComCFS_flg]
  [task_time_s] -> Gain1/1
  Gain1/1 -> Timer1/3
  [VINP_ADASISASta_enum] -> Equal1/1
  Equal1/1 -> Logical Operator1/3
  Equal9/1 -> Logical Operator10/2
  Constant3/1 -> Equal9/2
  Constant17/1 -> Equal1/2
  Equal11/1 -> Logical Operator13/2
  Logical Operator13/1 -> Logical Operator11/2
  Constant1/1 -> Equal8/2
  [VPMM_PowerSta_enum] -> Equal11/1
  [VINP_ADASACCSta_enum] -> Equal9/1
  [VINP_ADASACCSta_enum] -> Equal8/1
  Logical Operator1/1 -> Logical Operator11/1
  Constant8/1 -> Equal10/2
  [DTC_clear_request] -> Logical Operator11/3
  Equal10/1 -> Logical Operator13/1
  Logical Operator10/1 -> Logical Operator1/2
  Equal8/1 -> Logical Operator10/1
  [VPMM_PowerSta_enum] -> Unit Delay1/1
  Unit Delay1/1 -> Equal10/1
  Constant16/1 -> Equal11/2
  Logical Operator11/1 -> Switch4/2
  VINP_ADASISASta_enum/1 -> [VINP_ADASISASta_enum]
  [DTC_clear_request] -> Switch5/2
  Constant10/1 -> Switch5/1
  Switch5/1 -> Test Detection Criteria/1
  [VDDM_FCM3CSErrDet_flg] -> DTC_Info/1
  [VDDM_FCM3CSErrPass_flg] -> DTC_Info/2
  [VDDM_FCM3CSErrCFS_flg] -> DTC_Info/3
  [DTC_clear_request] -> DTC_Info/4
  DTC_Info/1 -> VDDM_FCM3CSErrDTC_raw32/1  "VDDM_FCM3CSErrDTC_raw32"

== system ddm/DDM/DDM/VMC_DDM/FCM3/FCM3 Lost Com ==
  note: Fail Safe After Decision
  note: Release Condiction During Detection
  note: Diagnostics and Fault Handling
  note: Test Pass Criteria
  note: Release Condiction After Decision
  note: Test Detection Criteria
  note: Fail Safe During Detection
  task_time_s : Inport
  VDDM_FCM3NoCom_flg : Inport  Port=2
  No_CAN_BUS_OFF : Inport  Port=3
  VPMM_PowerSta_enum : Inport  Port=4
  VINP_ADASACCSta_enum : Inport  Port=5
  VINP_ADASISASta_enum : Inport  Port=6
  DTC_clear_request : Inport  Port=7
  Constant : Constant  Value=ENUM_POWERSTA_OFF
  Constant{1..2,15,21,23} (5 alike) : Constant  Value=FALSE
  Constant10 : Constant  Value=ENUM_ADASACCSTA_OFF
  Constant11 : Constant  Value=ENUM_ADASACCSTA_STANDBY
  Constant12 : Constant  Value=ENUM_POWERSTA_OFF
  Constant13 : Constant  Value=ENUM_POWERSTA_STANDBY
  Constant{7,14,18,22} (4 alike) : Constant  Value=TRUE
  Constant3 : Constant  Value=ENUM_ADASISASTA_OFF
  Constant31 : Constant  Value=KDDM_FCM3NoComDFSSW_flg
  Constant4 : Constant  Value=KDDM_FCM3NoComCFSSW_flg
  Constant40 : Constant  Value=KDDM_FCM3NoComDTC_cnt
  Constant41 : Constant  Value=KDDM_FCM3NoComDetTO_ms
  Constant45 : Constant  Value=KDDM_FCM3NoComPassSW_flg
  Constant46 : Constant  Value=KDDM_FCM3NoComDetSW_flg
  Constant48 : Constant  Value=KDDM_FCM3NoComDTC_cnt
  Constant5 : Constant  Value=ENUM_POWERSTA_OFF
  Constant6 : Constant  Value=KDDM_FCM3NoComPassTO_ms
  Constant9 : Constant  Value=KDDM_FCM3NoComPassTO_ms
  DTC_Couter : hcu_lib/Basic_Blocks/DTC_Couter
  DTC_Info : hcu_lib/Basic_Blocks/DTC_Info
  Data Type Conversion1 : DataTypeConversion  OutDataTypeStr=uint8
  Display : Display
  Display1 : Display
  Display2 : Display
  Equal : RelationalOperator  Operator=~=  OutDataTypeStr=boolean  RndMeth=Simplest
  Equal{1,4..7} (5 alike) : RelationalOperator  Operator===  OutDataTypeStr=boolean  RndMeth=Simplest
  Equal2 : RelationalOperator  Operator=~=  OutDataTypeStr=boolean  RndMeth=Simplest
  Equal3 : RelationalOperator  OutDataTypeStr=boolean  RndMeth=Simplest
  From6 : From  Commented=on  GotoTag=VDDM_EDriveSysErrVCUErr_flg
  Gain : Gain  Gain=XX2KXX
  Gain1 : Gain  Gain=KXX2XX
  Goto7 : Goto  Commented=on  GotoTag=VDDM_EDriveSysErrVCUErr_flg
  Logical Operator{2,4,9,12,15,18..19} (7 alike) : Logic  AllPortsSameDT=off  OutDataTypeStr=boolean
  Logical Operator21 : Logic  Operator=OR  AllPortsSameDT=off  OutDataTypeStr=boolean
  Logical Operator3 : Logic  Operator=OR  AllPortsSameDT=off  OutDataTypeStr=boolean
  Logical Operator5 : Logic  Inputs=3  AllPortsSameDT=off  OutDataTypeStr=boolean
  Logical Operator6 : Logic  Operator=NOT  AllPortsSameDT=off  OutDataTypeStr=boolean
  Logical Operator7 : Logic  Operator=OR  AllPortsSameDT=off  OutDataTypeStr=boolean
  Logical Operator8 : Logic  Operator=OR  Inputs=3  AllPortsSameDT=off  OutDataTypeStr=boolean
  Relay : Relay  OnSwitchValue=ONE_INT  OffSwitchValue=ZERO_INT
  SR_Latch1 : hcu_lib/Basic_Blocks/SR_Latch
  SR_Latch3 : hcu_lib/Basic_Blocks/SR_Latch
  SR_Latch4 : hcu_lib/Basic_Blocks/SR_Latch
  Switch{,1..5} (6 alike) : Switch  Criteria=u2 ~= 0
  Terminator : Terminator
  Test Detection Criteria : hcu_lib/Basic_Blocks/Test Detection Criteria
  Timer1 : hcu_lib/Basic_Blocks/Timer
  Unit Delay2 : UnitDelay  SampleTime=-1  HasFrameUpgradeWarning=on
  VDDM_FCM3NoComDFS_flg : Outport
  VDDM_FCM3NoComCFS_flg : Outport  Port=2
  VDDM_FCM3NoComDTC_raw32 : Outport  Port=3
  wires:
  VPMM_PowerSta_enum/1 -> [VPMM_PowerSta_enum]
  DTC_clear_request/1 -> [DTC_clear_request]
  No_CAN_BUS_OFF/1 -> [No_CAN_BUS_OFF]
  VINP_ADASACCSta_enum/1 -> [VINP_ADASACCSta_enum]
  VDDM_FCM3NoCom_flg/1 -> [VDDM_FCM3NoCom_flg]
  [VDDM_FCM3NoComCFS_flg] -> VDDM_FCM3NoComCFS_flg/1
  [VDDM_FCM3NoComDFS_flg] -> VDDM_FCM3NoComDFS_flg/1
  From6/1 -> Terminator/1
  Logical Operator6/1 -> Timer1/1
  Logical Operator21/1 -> SR_Latch3/2
  [VDDM_FCM3NoComCFS_flg] -> Logical Operator21/2
  Constant22/1 -> Switch1/1
  [VDDM_xxx_flg] -> SR_Latch1/2
  [No_CAN_BUS_OFF] -> Logical Operator2/1
  [VDDM_FCM3NoComCFS_flg] -> Switch/2
  [VINP_ADASACCSta_enum] -> Equal4/1
  [VPMM_PowerSta_enum] -> Unit Delay2/1
  Constant15/1 -> Switch4/3
  [VDDM_FCM3NoComDTC_cnt] -> Relay/1
  [task_time_s] -> Gain1/1
  Equal6/1 -> Logical Operator9/1
  Constant13/1 -> Equal7/2
  Constant18/1 -> Switch/1
  Equal3/1 -> SR_Latch1/1
  Switch1/1 -> [VDDM_FCM3NoComDFSRls_flg]
  Switch/1 -> Display1/1, Goto7/1
  Constant5/1 -> Equal2/2
  [DTC_clear_request] -> Logical Operator8/3
  Unit Delay2/1 -> Equal6/1
  Constant12/1 -> Equal6/2
  Constant2/1 -> Switch2/3
  Logical Operator7/1 -> Logical Operator5/2
  Constant14/1 -> Switch4/1
  Logical Operator4/1 -> Switch3/2
  Equal4/1 -> Logical Operator7/1
  Equal5/1 -> Logical Operator7/2
  Constant7/1 -> Switch3/3
  Logical Operator5/1 -> Logical Operator8/1
  Constant4/1 -> Logical Operator18/2
  [VDDM_FCM3NoCom_flg] -> Switch2/1
  Equal7/1 -> Logical Operator9/2
  [VDDM_FCM3NoComCFSRls_flg] -> Logical Operator3/2
  Data Type Conversion1/1 -> [VDDM_FCM3NoComDTC_cnt]
  Constant21/1 -> Switch/3
  [VDDM_FCM3NoComCFSRls_flg] -> SR_Latch4/2
  Constant31/1 -> Logical Operator12/1
  [VDDM_FCM3NoComPass_flg] -> Switch1/2
  Timer1/1 -> Equal3/1
  Constant23/1 -> Switch1/3
  [VDDM_FCM3NoComDet_flg] -> Logical Operator19/1
  SR_Latch4/1 -> Logical Operator18/1
  Logical Operator2/1 -> Switch2/2
  Test Detection Criteria/1 -> [VDDM_FCM3NoComDet_flg]
  [task_time_s] -> Test Detection Criteria/2
  Constant46/1 -> Logical Operator19/2
  [VINP_ADASACCSta_enum] -> Equal5/1
  Logical Operator12/1 -> [VDDM_FCM3NoComDFS_flg]
  Constant41/1 -> Gain/1
  [VDDM_FCM3NoComDFSRls_flg] -> Logical Operator21/1
  Switch4/1 -> Display2/1, [VDDM_FCM3NoComCFSRls_flg]
  Constant11/1 -> Equal5/2
  [VPMM_PowerSta_enum] -> Equal/1
  Switch3/1 -> Logical Operator6/1, Timer1/2
  Constant/1 -> Equal/2
  DTC_Couter/1 -> SR_Latch4/1
  [VDDM_FCM3NoComPass_flg] -> Logical Operator3/1
  Constant45/1 -> Logical Operator15/2
  Logical Operator19/1 -> DTC_Couter/1
  [VDDM_FCM3NoCom_flg] -> Switch3/1
  [VPMM_PowerSta_enum] -> Equal2/1
  [VPMM_PowerSta_enum] -> Equal7/1
  Logical Operator8/1 -> Switch4/2
  Logical Operator9/1 -> Logical Operator8/2
  [No_CAN_BUS_OFF] -> Logical Operator4/1
  Constant10/1 -> Equal4/2
  Constant48/1 -> DTC_Couter/3
  Equal2/1 -> Logical Operator4/2
  [VDDM_FCM3NoComPass_flg] -> Logical Operator5/1
  Logical Operator3/1 -> Logical Operator15/1
  Relay/1 -> SR_Latch3/1
  Logical Operator18/1 -> [VDDM_FCM3NoComCFS_flg]
  Equal/1 -> Logical Operator2/2
  Gain/1 -> Test Detection Criteria/4
  SR_Latch1/1 -> Display/1, [VDDM_FCM3NoComPass_flg]
  Constant6/1 -> Equal3/2
  Logical Operator15/1 -> DTC_Couter/2
  SR_Latch3/1 -> Logical Operator12/2
  Constant40/1 -> Test Detection Criteria/3
  DTC_Couter/2 -> Data Type Conversion1/1
  task_time_s/1 -> [task_time_s]  "task_time_s"
  Constant9/1 -> Timer1/4
  Gain1/1 -> Timer1/3
  Constant3/1 -> Equal1/2
  [VINP_ADASISASta_enum] -> Equal1/1
  Equal1/1 -> Logical Operator5/3
  VINP_ADASISASta_enum/1 -> [VINP_ADASISASta_enum]
  Switch2/1 -> [VDDM_xxx_flg], Switch5/3
  Constant1/1 -> Switch5/1
  [DTC_clear_request] -> Switch5/2
  Switch5/1 -> Test Detection Criteria/1
  [VDDM_FCM3NoComDet_flg] -> DTC_Info/1
  [VDDM_FCM3NoComPass_flg] -> DTC_Info/2
  [VDDM_FCM3NoComCFS_flg] -> DTC_Info/3
  [DTC_clear_request] -> DTC_Info/4
  DTC_Info/1 -> VDDM_FCM3NoComDTC_raw32/1  "VDDM_FCM3NoComDTC_raw32"
